simulink model "EMB_LRM"  (R2025a)
settings: Solver=FixedStepDiscrete  StartTime=0.0  StopTime=100  FixedStep=0.01  RelTol=1e-3
settings Model: Creator=wangtianqi  LastModifiedBy=wangtianqi

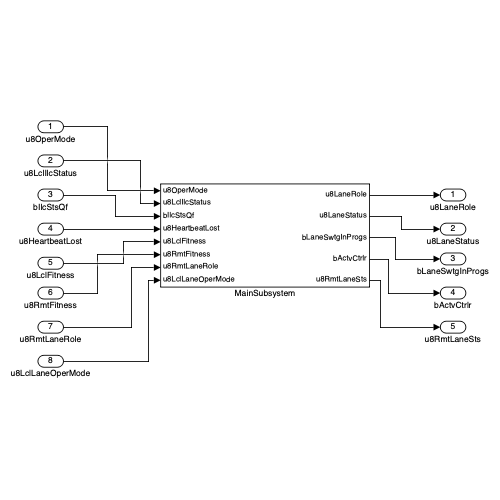
[thumbnail: Simulink's stored preview of the top-level diagram]
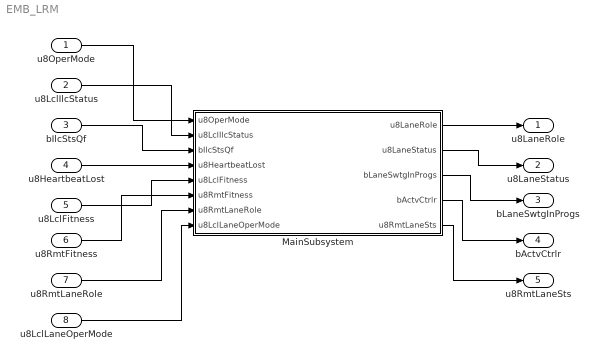
== system EMB_LRM ==
  u8OperMode : Inport  Description=系统运行模式: 0=INIT,1=NORMAL_OPERATION,2=LIMP_HOME,3=LIMP_ASIDE,4=CRAWL,5=SHUTTING_DOWN  OutMin=0  OutMax=5  OutDataTypeStr=uint8
  u8LclIlcStatus : Inport  Description=本控制链路ILC状态: 0=Failed,1=Normal,2=Initialized  Port=2  OutMin=0  OutMax=2  OutDataTypeStr=uint8
  bIlcStsQf : Inport  Description=ILC状态信号质量: 0=QF_Full,1=QF_NotFull  Port=3  OutMin=0  OutMax=1  OutDataTypeStr=boolean
  u8HeartbeatLost : Inport  Description=心跳丢失计数  Port=4  OutMin=0  OutMax=255  OutDataTypeStr=uint8
  u8LclFitness : Inport  Description=本控制链路健康度得分(62=禁用,255=无效)  Port=5  OutMin=0  OutMax=255  OutDataTypeStr=uint8
  u8RmtFitness : Inport  Description=远控制链路健康度得分(62=禁用,255=无效)  Port=6  OutMin=0  OutMax=255  OutDataTypeStr=uint8
  u8RmtLaneRole : Inport  Description=远控制链路角色: 0=INIT,1=MASTER,2=FALLBACK,3=SUPPORT,4=DISABLED,5=SHUTTING_DOWN  Port=7  OutMin=0  OutMax=5  OutDataTypeStr=uint8
  u8LclLaneOperMode : Inport  Description=本控制链路运行模式: 0=INIT,1=NORMAL_OPERATION,2=LIMP_HOME,3=LIMP_ASIDE,4=CRAWL,5=SHUTTING_DOWN  Port=8  OutMin=0  OutMax=5  OutDataTypeStr=uint8
  MainSubsystem : Subsystem  Description=主功能包装层：信号调理 → 功能模块 → 输出仲裁
  u8LaneRole : Outport  Description=本控制链路角色: 0=UNKNOWN,1=INIT,2=MASTER,3=FALLBACK,4=SUPPORT,5=DISABLED,6=SHUTTING_DOWN  OutMin=0  OutMax=6  OutDataTypeStr=uint8
  u8LaneStatus : Outport  Description=控制链路状态: 0=INITIALISING,1=OPERATING,2=HB_LOST,3=FAILED  Port=2  OutMin=0  OutMax=3  OutDataTypeStr=uint8
  bLaneSwtgInProgs : Outport  Description=控制链路切换进行中: 0=NotProgress,1=Progress  Port=3  OutMin=0  OutMax=1  OutDataTypeStr=boolean
  bActvCtrlr : Outport  Description=活动控制器实例: 0=NotActive,1=Active  Port=4  OutMin=0  OutMax=1  OutDataTypeStr=boolean
  u8RmtLaneSts : Outport  Description=远控制链路状态: 0=INITIALISING,1=OPERATING,2=HB_LOST,3=FAILED  Port=5  OutMin=0  OutMax=3  OutDataTypeStr=uint8
  wires:
  MainSubsystem/5(u8RmtLaneSts) -> u8RmtLaneSts/1
  u8OperMode/1 -> MainSubsystem/1(u8OperMode)
  MainSubsystem/3(bLaneSwtgInProgs) -> bLaneSwtgInProgs/1
  MainSubsystem/1(u8LaneRole) -> u8LaneRole/1
  u8RmtFitness/1 -> MainSubsystem/6(u8RmtFitness)
  u8LclLaneOperMode/1 -> MainSubsystem/8(u8LclLaneOperMode)
  u8LclFitness/1 -> MainSubsystem/5(u8LclFitness)
  u8HeartbeatLost/1 -> MainSubsystem/4(u8HeartbeatLost)
  bIlcStsQf/1 -> MainSubsystem/3(bIlcStsQf)
  MainSubsystem/4(bActvCtrlr) -> bActvCtrlr/1
  MainSubsystem/2(u8LaneStatus) -> u8LaneStatus/1
  u8RmtLaneRole/1 -> MainSubsystem/7(u8RmtLaneRole)
  u8LclIlcStatus/1 -> MainSubsystem/2(u8LclIlcStatus)

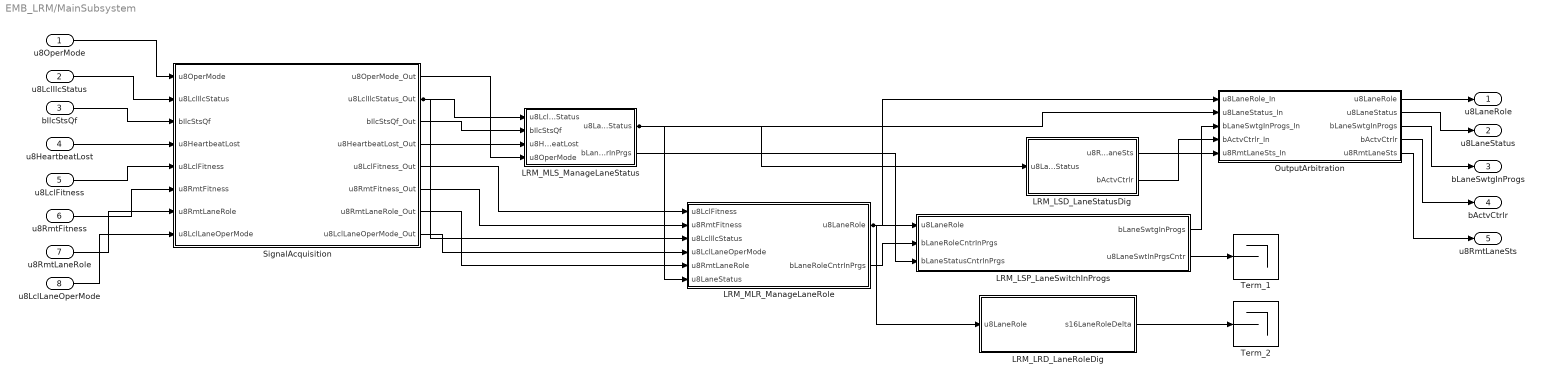
== system EMB_LRM/MainSubsystem ==
  u8OperMode : Inport
  u8LclIlcStatus : Inport  Port=2
  bIlcStsQf : Inport  Port=3
  u8HeartbeatLost : Inport  Port=4
  u8LclFitness : Inport  Port=5
  u8RmtFitness : Inport  Port=6
  u8RmtLaneRole : Inport  Port=7
  u8LclLaneOperMode : Inport  Port=8
  LRM_LRD_LaneRoleDig : Subsystem
  LRM_LSD_LaneStatusDig : Subsystem
  LRM_LSP_LaneSwitchInProgs : Subsystem
  LRM_MLR_ManageLaneRole : Subsystem
  LRM_MLS_ManageLaneStatus : Subsystem
  OutputArbitration : Subsystem
  SignalAcquisition : Subsystem
  Term_1 : Terminator
  Term_2 : Terminator
  u8LaneRole : Outport
  u8LaneStatus : Outport  Port=2
  bLaneSwtgInProgs : Outport  Port=3
  bActvCtrlr : Outport  Port=4
  u8RmtLaneSts : Outport  Port=5
  wires:
  OutputArbitration/5(u8RmtLaneSts) -> u8RmtLaneSts/1
  OutputArbitration/1(u8LaneRole) -> u8LaneRole/1
  LRM_LRD_LaneRoleDig/1(s16LaneRoleDelta) -> Term_2/1
  LRM_LSP_LaneSwitchInProgs/2(u8LaneSwtInPrgsCntr) -> Term_1/1
  SignalAcquisition/7(u8RmtLaneRole_Out) -> LRM_MLR_ManageLaneRole/5(u8RmtLaneRole)
  LRM_LSP_LaneSwitchInProgs/1(bLaneSwtgInProgs) -> OutputArbitration/3(bLaneSwtgInProgs_In)
  OutputArbitration/4(bActvCtrlr) -> bActvCtrlr/1
  LRM_MLS_ManageLaneStatus/2(bLaneStatusCntrInPrgs) -> LRM_LSP_LaneSwitchInProgs/3(bLaneStatusCntrInPrgs)
  SignalAcquisition/8(u8LclLaneOperMode_Out) -> LRM_MLR_ManageLaneRole/4(u8LclLaneOperMode)
  OutputArbitration/3(bLaneSwtgInProgs) -> bLaneSwtgInProgs/1
  LRM_MLS_ManageLaneStatus/1(u8LaneStatus) -> LRM_MLR_ManageLaneRole/6(u8LaneStatus), LRM_LSD_LaneStatusDig/1(u8LaneStatus), OutputArbitration/2(u8LaneStatus_In)
  u8RmtLaneRole/1 -> SignalAcquisition/7(u8RmtLaneRole)
  LRM_LSD_LaneStatusDig/2(bActvCtrlr) -> OutputArbitration/4(bActvCtrlr_In)
  SignalAcquisition/6(u8RmtFitness_Out) -> LRM_MLR_ManageLaneRole/2(u8RmtFitness)
  LRM_MLR_ManageLaneRole/2(bLaneRoleCntrInPrgs) -> LRM_LSP_LaneSwitchInProgs/2(bLaneRoleCntrInPrgs)
  SignalAcquisition/5(u8LclFitness_Out) -> LRM_MLR_ManageLaneRole/1(u8LclFitness)
  SignalAcquisition/3(bIlcStsQf_Out) -> LRM_MLS_ManageLaneStatus/2(bIlcStsQf)
  SignalAcquisition/2(u8LclIlcStatus_Out) -> LRM_MLS_ManageLaneStatus/1(u8LclIlcStatus), LRM_MLR_ManageLaneRole/3(u8LclIlcStatus)
  LRM_LSD_LaneStatusDig/1(u8RmtLaneSts) -> OutputArbitration/5(u8RmtLaneSts_In)
  u8LclLaneOperMode/1 -> SignalAcquisition/8(u8LclLaneOperMode)
  u8RmtFitness/1 -> SignalAcquisition/6(u8RmtFitness)
  SignalAcquisition/1(u8OperMode_Out) -> LRM_MLS_ManageLaneStatus/4(u8OperMode)
  u8LclFitness/1 -> SignalAcquisition/5(u8LclFitness)
  u8LclIlcStatus/1 -> SignalAcquisition/2(u8LclIlcStatus)
  OutputArbitration/2(u8LaneStatus) -> u8LaneStatus/1
  u8HeartbeatLost/1 -> SignalAcquisition/4(u8HeartbeatLost)
  bIlcStsQf/1 -> SignalAcquisition/3(bIlcStsQf)
  LRM_MLR_ManageLaneRole/1(u8LaneRole) -> LRM_LRD_LaneRoleDig/1(u8LaneRole), LRM_LSP_LaneSwitchInProgs/1(u8LaneRole), OutputArbitration/1(u8LaneRole_In)
  SignalAcquisition/4(u8HeartbeatLost_Out) -> LRM_MLS_ManageLaneStatus/3(u8HeartbeatLost)
  u8OperMode/1 -> SignalAcquisition/1(u8OperMode)

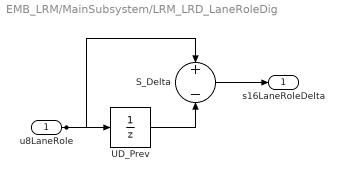
== system EMB_LRM/MainSubsystem/LRM_LRD_LaneRoleDig ==
  u8LaneRole : Inport
  S_Delta : Sum  Inputs=+-
  UD_Prev : UnitDelay
  s16LaneRoleDelta : Outport
  wires:
  S_Delta/1 -> s16LaneRoleDelta/1
  UD_Prev/1 -> S_Delta/2
  u8LaneRole/1 -> UD_Prev/1, S_Delta/1

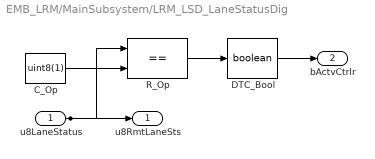
== system EMB_LRM/MainSubsystem/LRM_LSD_LaneStatusDig ==
  u8LaneStatus : Inport
  C_Op : Constant  Value=uint8(1)
  DTC_Bool : DataTypeConversion  OutDataTypeStr=boolean
  R_Op : RelationalOperator  Operator===
  u8RmtLaneSts : Outport
  bActvCtrlr : Outport  Port=2
  wires:
  DTC_Bool/1 -> bActvCtrlr/1
  R_Op/1 -> DTC_Bool/1
  u8LaneStatus/1 -> u8RmtLaneSts/1, R_Op/1
  C_Op/1 -> R_Op/2

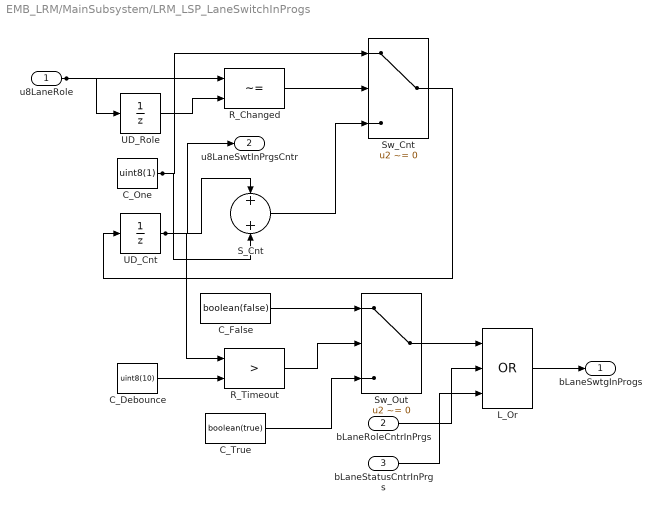
== system EMB_LRM/MainSubsystem/LRM_LSP_LaneSwitchInProgs ==
  u8LaneRole : Inport
  bLaneRoleCntrInPrgs : Inport  Port=2
  bLaneStatusCntrInPrgs : Inport  Port=3
  C_Debounce : Constant  Value=uint8(10)
  C_False : Constant  Value=boolean(false)
  C_One : Constant  Value=uint8(1)
  C_True : Constant  Value=boolean(true)
  L_Or : Logic  Operator=OR  Inputs=3  AllPortsSameDT=off  OutDataTypeStr=boolean
  R_Changed : RelationalOperator  Operator=~=
  R_Timeout : RelationalOperator  Operator=>
  S_Cnt : Sum
  Sw_Cnt : Switch  Criteria=u2 ~= 0
  Sw_Out : Switch  Criteria=u2 ~= 0
  UD_Cnt : UnitDelay
  UD_Role : UnitDelay
  bLaneSwtgInProgs : Outport
  u8LaneSwtInPrgsCntr : Outport  Port=2
  wires:
  bLaneRoleCntrInPrgs/1 -> L_Or/2
  Sw_Out/1 -> L_Or/1
  bLaneStatusCntrInPrgs/1 -> L_Or/3
  S_Cnt/1 -> Sw_Cnt/3
  R_Timeout/1 -> Sw_Out/2
  C_One/1 -> Sw_Cnt/1, S_Cnt/2
  C_False/1 -> Sw_Out/1
  L_Or/1 -> bLaneSwtgInProgs/1
  UD_Cnt/1 -> u8LaneSwtInPrgsCntr/1, R_Timeout/1, S_Cnt/1
  C_Debounce/1 -> R_Timeout/2
  Sw_Cnt/1 -> UD_Cnt/1
  C_True/1 -> Sw_Out/3
  R_Changed/1 -> Sw_Cnt/2
  UD_Role/1 -> R_Changed/2
  u8LaneRole/1 -> UD_Role/1, R_Changed/1

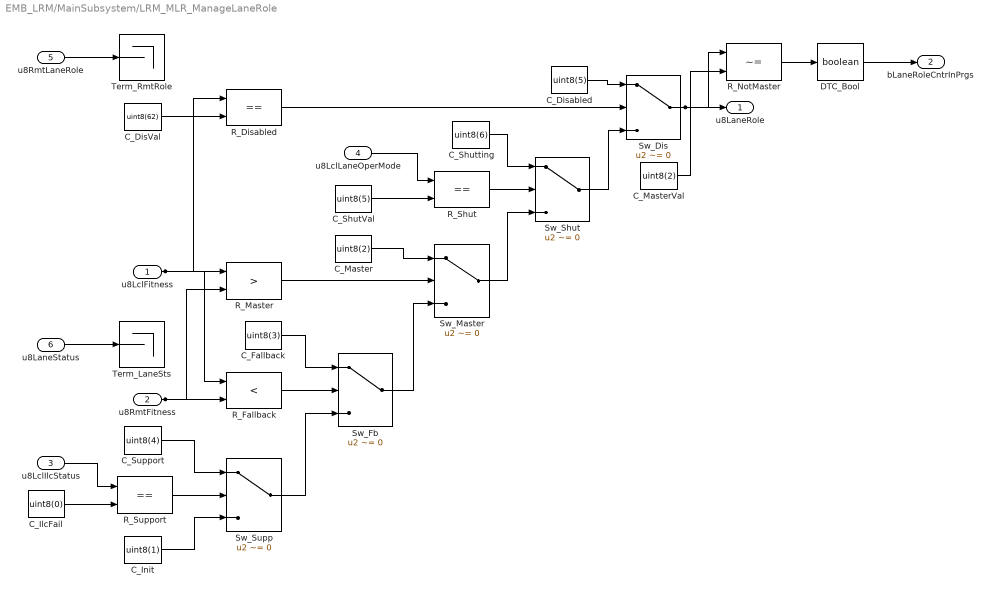
== system EMB_LRM/MainSubsystem/LRM_MLR_ManageLaneRole ==
  u8LclFitness : Inport
  u8RmtFitness : Inport  Port=2
  u8LclIlcStatus : Inport  Port=3
  u8LclLaneOperMode : Inport  Port=4
  u8RmtLaneRole : Inport  Port=5
  u8LaneStatus : Inport  Port=6
  C_DisVal : Constant  Value=uint8(62)
  C_Disabled : Constant  Value=uint8(5)
  C_Fallback : Constant  Value=uint8(3)
  C_IlcFail : Constant  Value=uint8(0)
  C_Init : Constant  Value=uint8(1)
  C_Master : Constant  Value=uint8(2)
  C_MasterVal : Constant  Value=uint8(2)
  C_ShutVal : Constant  Value=uint8(5)
  C_Shutting : Constant  Value=uint8(6)
  C_Support : Constant  Value=uint8(4)
  DTC_Bool : DataTypeConversion  OutDataTypeStr=boolean
  R_Disabled : RelationalOperator  Operator===
  R_Fallback : RelationalOperator  Operator=<
  R_Master : RelationalOperator  Operator=>
  R_NotMaster : RelationalOperator  Operator=~=
  R_Shut : RelationalOperator  Operator===
  R_Support : RelationalOperator  Operator===
  Sw_Dis : Switch  Criteria=u2 ~= 0
  Sw_Fb : Switch  Criteria=u2 ~= 0
  Sw_Master : Switch  Criteria=u2 ~= 0
  Sw_Shut : Switch  Criteria=u2 ~= 0
  Sw_Supp : Switch  Criteria=u2 ~= 0
  Term_LaneSts : Terminator
  Term_RmtRole : Terminator
  u8LaneRole : Outport
  bLaneRoleCntrInPrgs : Outport  Port=2
  wires:
  DTC_Bool/1 -> bLaneRoleCntrInPrgs/1
  C_MasterVal/1 -> R_NotMaster/2
  Sw_Dis/1 -> R_NotMaster/1, u8LaneRole/1
  Sw_Shut/1 -> Sw_Dis/3
  u8LaneStatus/1 -> Term_LaneSts/1
  Sw_Master/1 -> Sw_Shut/3
  C_Master/1 -> Sw_Master/1
  C_ShutVal/1 -> R_Shut/2
  C_Disabled/1 -> Sw_Dis/1
  R_Shut/1 -> Sw_Shut/2
  R_Fallback/1 -> Sw_Fb/2
  C_Support/1 -> Sw_Supp/1
  u8RmtFitness/1 -> R_Fallback/2, R_Master/2
  C_Fallback/1 -> Sw_Fb/1
  R_Disabled/1 -> Sw_Dis/2
  u8LclFitness/1 -> R_Fallback/1, R_Master/1, R_Disabled/1
  C_Shutting/1 -> Sw_Shut/1
  u8RmtLaneRole/1 -> Term_RmtRole/1
  R_NotMaster/1 -> DTC_Bool/1
  R_Support/1 -> Sw_Supp/2
  C_Init/1 -> Sw_Supp/3
  Sw_Supp/1 -> Sw_Fb/3
  u8LclLaneOperMode/1 -> R_Shut/1
  u8LclIlcStatus/1 -> R_Support/1
  C_DisVal/1 -> R_Disabled/2
  R_Master/1 -> Sw_Master/2
  C_IlcFail/1 -> R_Support/2
  Sw_Fb/1 -> Sw_Master/3

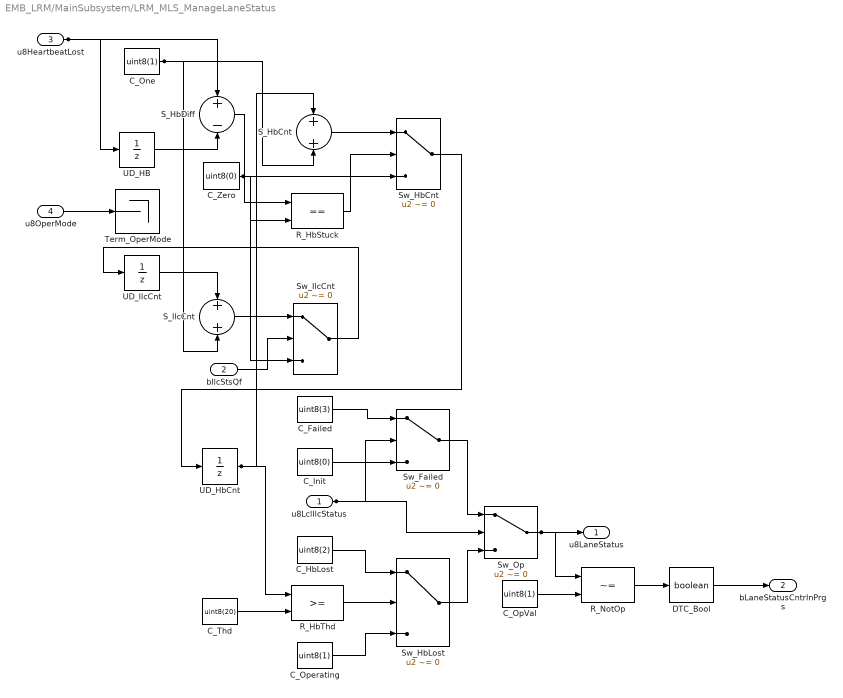
== system EMB_LRM/MainSubsystem/LRM_MLS_ManageLaneStatus ==
  u8LclIlcStatus : Inport
  bIlcStsQf : Inport  Port=2
  u8HeartbeatLost : Inport  Port=3
  u8OperMode : Inport  Port=4
  C_Failed : Constant  Value=uint8(3)
  C_HbLost : Constant  Value=uint8(2)
  C_Init : Constant  Value=uint8(0)
  C_One : Constant  Value=uint8(1)
  C_OpVal : Constant  Value=uint8(1)
  C_Operating : Constant  Value=uint8(1)
  C_Thd : Constant  Value=uint8(20)
  C_Zero : Constant  Value=uint8(0)
  DTC_Bool : DataTypeConversion  OutDataTypeStr=boolean
  R_HbStuck : RelationalOperator  Operator===
  R_HbThd : RelationalOperator
  R_NotOp : RelationalOperator  Operator=~=
  S_HbCnt : Sum
  S_HbDiff : Sum  Inputs=+-
  S_IlcCnt : Sum
  Sw_Failed : Switch  Criteria=u2 ~= 0
  Sw_HbCnt : Switch  Criteria=u2 ~= 0
  Sw_HbLost : Switch  Criteria=u2 ~= 0
  Sw_IlcCnt : Switch  Criteria=u2 ~= 0
  Sw_Op : Switch  Criteria=u2 ~= 0
  Term_OperMode : Terminator
  UD_HB : UnitDelay
  UD_HbCnt : UnitDelay
  UD_IlcCnt : UnitDelay
  u8LaneStatus : Outport
  bLaneStatusCntrInPrgs : Outport  Port=2
  wires:
  DTC_Bool/1 -> bLaneStatusCntrInPrgs/1
  R_NotOp/1 -> DTC_Bool/1
  C_OpVal/1 -> R_NotOp/2
  Sw_Op/1 -> R_NotOp/1, u8LaneStatus/1
  Sw_HbCnt/1 -> UD_HbCnt/1
  C_Init/1 -> Sw_Failed/3
  Sw_Failed/1 -> Sw_Op/1
  C_Failed/1 -> Sw_Failed/1
  u8LclIlcStatus/1 -> Sw_Failed/2, Sw_Op/2
  C_Zero/1 -> Sw_IlcCnt/3, R_HbStuck/2, Sw_HbCnt/3
  Sw_IlcCnt/1 -> UD_IlcCnt/1
  Sw_HbLost/1 -> Sw_Op/3
  C_Operating/1 -> Sw_HbLost/3
  S_HbCnt/1 -> Sw_HbCnt/1
  C_Thd/1 -> R_HbThd/2
  UD_HbCnt/1 -> R_HbThd/1, S_HbCnt/1
  bIlcStsQf/1 -> Sw_IlcCnt/2
  S_IlcCnt/1 -> Sw_IlcCnt/1
  S_HbDiff/1 -> R_HbStuck/1
  UD_IlcCnt/1 -> S_IlcCnt/1
  R_HbStuck/1 -> Sw_HbCnt/2
  u8OperMode/1 -> Term_OperMode/1
  R_HbThd/1 -> Sw_HbLost/2
  C_HbLost/1 -> Sw_HbLost/1
  UD_HB/1 -> S_HbDiff/2
  C_One/1 -> S_HbCnt/2, S_IlcCnt/2
  u8HeartbeatLost/1 -> UD_HB/1, S_HbDiff/1

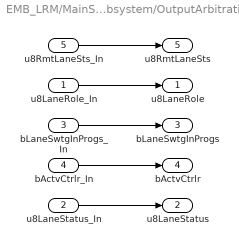
== system EMB_LRM/MainSubsystem/OutputArbitration ==
  u8LaneRole_In : Inport
  u8LaneStatus_In : Inport  Port=2
  bLaneSwtgInProgs_In : Inport  Port=3
  bActvCtrlr_In : Inport  Port=4
  u8RmtLaneSts_In : Inport  Port=5
  u8LaneRole : Outport
  u8LaneStatus : Outport  Port=2
  bLaneSwtgInProgs : Outport  Port=3
  bActvCtrlr : Outport  Port=4
  u8RmtLaneSts : Outport  Port=5
  wires:
  u8LaneStatus_In/1 -> u8LaneStatus/1
  bActvCtrlr_In/1 -> bActvCtrlr/1
  bLaneSwtgInProgs_In/1 -> bLaneSwtgInProgs/1
  u8LaneRole_In/1 -> u8LaneRole/1
  u8RmtLaneSts_In/1 -> u8RmtLaneSts/1

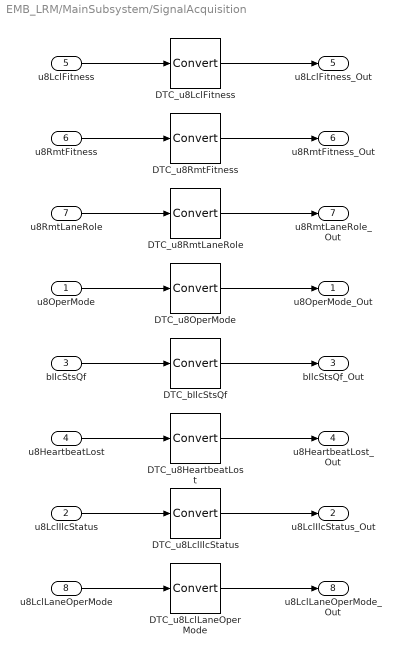
== system EMB_LRM/MainSubsystem/SignalAcquisition ==
  u8OperMode : Inport
  u8LclIlcStatus : Inport  Port=2
  bIlcStsQf : Inport  Port=3
  u8HeartbeatLost : Inport  Port=4
  u8LclFitness : Inport  Port=5
  u8RmtFitness : Inport  Port=6
  u8RmtLaneRole : Inport  Port=7
  u8LclLaneOperMode : Inport  Port=8
  DTC_bIlcStsQf : DataTypeConversion
  DTC_u8HeartbeatLost : DataTypeConversion
  DTC_u8LclFitness : DataTypeConversion
  DTC_u8LclIlcStatus : DataTypeConversion
  DTC_u8LclLaneOperMode : DataTypeConversion
  DTC_u8OperMode : DataTypeConversion
  DTC_u8RmtFitness : DataTypeConversion
  DTC_u8RmtLaneRole : DataTypeConversion
  u8OperMode_Out : Outport
  u8LclIlcStatus_Out : Outport  Port=2
  bIlcStsQf_Out : Outport  Port=3
  u8HeartbeatLost_Out : Outport  Port=4
  u8LclFitness_Out : Outport  Port=5
  u8RmtFitness_Out : Outport  Port=6
  u8RmtLaneRole_Out : Outport  Port=7
  u8LclLaneOperMode_Out : Outport  Port=8
  wires:
  DTC_u8LclIlcStatus/1 -> u8LclIlcStatus_Out/1
  DTC_u8HeartbeatLost/1 -> u8HeartbeatLost_Out/1
  DTC_bIlcStsQf/1 -> bIlcStsQf_Out/1
  DTC_u8OperMode/1 -> u8OperMode_Out/1
  DTC_u8RmtLaneRole/1 -> u8RmtLaneRole_Out/1
  u8LclLaneOperMode/1 -> DTC_u8LclLaneOperMode/1
  u8RmtLaneRole/1 -> DTC_u8RmtLaneRole/1
  DTC_u8RmtFitness/1 -> u8RmtFitness_Out/1
  u8LclIlcStatus/1 -> DTC_u8LclIlcStatus/1
  DTC_u8LclLaneOperMode/1 -> u8LclLaneOperMode_Out/1
  u8HeartbeatLost/1 -> DTC_u8HeartbeatLost/1
  bIlcStsQf/1 -> DTC_bIlcStsQf/1
  DTC_u8LclFitness/1 -> u8LclFitness_Out/1
  u8OperMode/1 -> DTC_u8OperMode/1
  u8RmtFitness/1 -> DTC_u8RmtFitness/1
  u8LclFitness/1 -> DTC_u8LclFitness/1
